simulink model "Motor_Pos_cl"  (R2015a)
settings: Solver=ode15s  StartTime=0.0  StopTime=10  RelTol=1e-3
values from neighbouring files (symbols this model uses):
  b = 3.5077E-6    (= 3.5077e-06)    [Motor_Pos_cl_m.m]
  J = 3.2284E-6    (= 3.2284e-06)    [Motor_Pos_cl_m.m]
  K = 0.0274    [Motor_Pos_cl_m.m]
  kd = 0    [Motor_Pos_cl_m.m]
  ki = 0    [Motor_Pos_cl_m.m]
  kp = 0.8    [Motor_Pos_cl_m.m]
  L = 2.75E-6    (= 2.75e-06)    [Motor_Pos_cl_m.m]
  R = 4    [Motor_Pos_cl_m.m]
  T1 = 0.040    (= 0.04)    [Motor_Pos_cl_m.m]
  T2 = 0.050    (= 0.05)    [Motor_Pos_cl_m.m]
libraries: simulink x2
settings Model: Creator=maen  LastModifiedBy=Xiaotian
settings DataIOCC: SignalLoggingSaveFormat=ModelDataLogs
settings OptimizationCC: ExpressionDepthLimit=2147483647
settings DebuggingCC: UnderspecifiedInitializationDetection=Classic  MergeDetectMultiDrivingBlocksExec=none  FcnCallInpInsideContextMsg=UseLocalSettings  StateNameClashWarn=warning
settings GRTTargetCC: CombineOutputUpdateFcns=off  GRTInterface=on

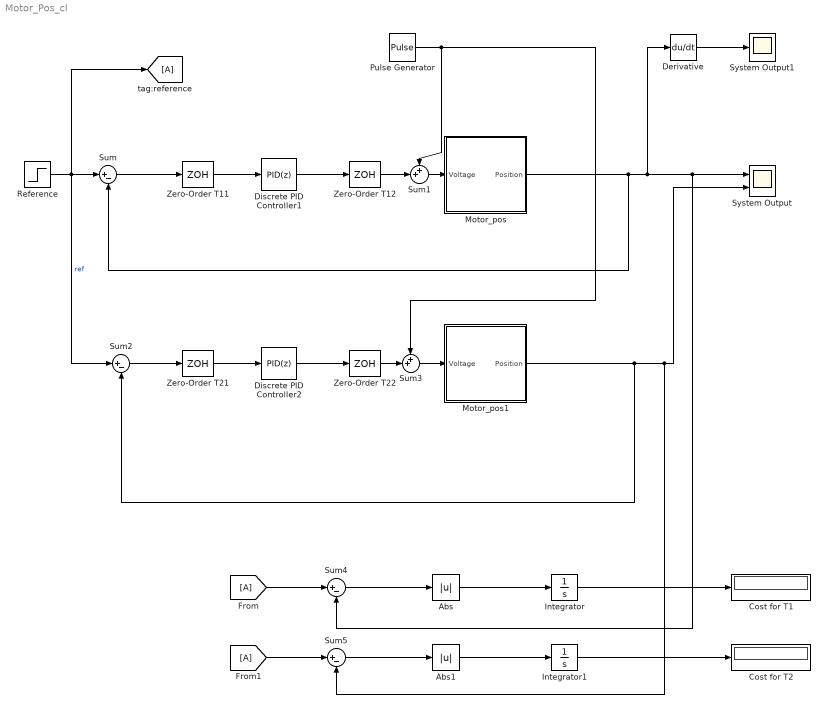
== system Motor_Pos_cl ==
  Abs : Abs
  Abs1 : Abs
  Cost for T1 : Display
  Cost for T2 : Display
  Derivative : Derivative
  Discrete PID Controller1 : simulink/Continuous/PID Controller  Controller=PID  TimeDomain=Discrete-time  SampleTime=T1  IntegratorMethod=Forward Euler  FilterMethod=Forward Euler  Form=Parallel  UseFilter=on  ControllerParametersSource=internal  P=kp  I=ki  D=kd  N=100  InitialConditionSource=internal  InitialConditionForIntegrator=0  InitialConditionForFilter=0  ExternalReset=none  LimitOutput=off  UpperSaturationLimit=inf  LowerSaturationLimit=-inf  LinearizeAsGain=off  AntiWindupMode=none  Kb=1  TrackingMode=off  Kt=1  PParamMin=[]  PParamMax=[]  IParamMin=[]  IParamMax=[]  DParamMin=[]  DParamMax=[]  NParamMin=[]  NParamMax=[]  KbParamMin=[]  KbParamMax=[]  KtParamMin=[]  KtParamMax=[]  POutMin=[]  POutMax=[]  IOutMin=[]  IOutMax=[]  DOutMin=[]  DOutMax=[]  NOutMin=[]  NOutMax=[]  KbOutMin=[]  KbOutMax=[]  KtOutMin=[]  KtOutMax=[]  IntegratorOutMin=[]  IntegratorOutMax=[]  FilterOutMin=[]  FilterOutMax=[]  SumOutMin=[]  SumOutMax=[]  SumI1OutMin=[]  SumI1OutMax=[]  SumI2OutMin=[]  SumI2OutMax=[]  SumI3OutMin=[]  SumI3OutMax=[]  SumDOutMin=[]  SumDOutMax=[]  SaturationOutMin=[]  SaturationOutMax=[]  IntegratorContinuousStateAttributes=''  IntegratorStateMustResolveToSignalObject=off  IntegratorRTWStateStorageClass=Auto  FilterContinuousStateAttributes=''  FilterStateMustResolveToSignalObject=off  FilterRTWStateStorageClass=Auto  DifferentiatorICPrevScaledInput=0  DifferentiatorOutMin=[]  DifferentiatorOutMax=[]
  Discrete PID Controller2 : simulink/Continuous/PID Controller  Controller=PID  TimeDomain=Discrete-time  SampleTime=T2  IntegratorMethod=Forward Euler  FilterMethod=Forward Euler  Form=Parallel  UseFilter=on  ControllerParametersSource=internal  P=kp  I=ki  D=kd  N=100  InitialConditionSource=internal  InitialConditionForIntegrator=0  InitialConditionForFilter=0  ExternalReset=none  LimitOutput=off  UpperSaturationLimit=inf  LowerSaturationLimit=-inf  LinearizeAsGain=off  AntiWindupMode=none  Kb=1  TrackingMode=off  Kt=1  PParamMin=[]  PParamMax=[]  IParamMin=[]  IParamMax=[]  DParamMin=[]  DParamMax=[]  NParamMin=[]  NParamMax=[]  KbParamMin=[]  KbParamMax=[]  KtParamMin=[]  KtParamMax=[]  POutMin=[]  POutMax=[]  IOutMin=[]  IOutMax=[]  DOutMin=[]  DOutMax=[]  NOutMin=[]  NOutMax=[]  KbOutMin=[]  KbOutMax=[]  KtOutMin=[]  KtOutMax=[]  IntegratorOutMin=[]  IntegratorOutMax=[]  FilterOutMin=[]  FilterOutMax=[]  SumOutMin=[]  SumOutMax=[]  SumI1OutMin=[]  SumI1OutMax=[]  SumI2OutMin=[]  SumI2OutMax=[]  SumI3OutMin=[]  SumI3OutMax=[]  SumDOutMin=[]  SumDOutMax=[]  SaturationOutMin=[]  SaturationOutMax=[]  IntegratorContinuousStateAttributes=''  IntegratorStateMustResolveToSignalObject=off  IntegratorRTWStateStorageClass=Auto  FilterContinuousStateAttributes=''  FilterStateMustResolveToSignalObject=off  FilterRTWStateStorageClass=Auto  DifferentiatorICPrevScaledInput=0  DifferentiatorOutMin=[]  DifferentiatorOutMax=[]
  Integrator : Integrator
  Integrator1 : Integrator
  Motor_pos : Subsystem
  Motor_pos1 : Subsystem
  Pulse Generator : DiscretePulseGenerator  PulseType=Time based  Amplitude=0.5  PulseWidth=2  PhaseDelay=2
  Reference : Step  Time=0  SampleTime=0
  Sum{,2,4..5} (4 alike) : Sum  Inputs=|+-
  Sum1 : Sum  Inputs=++|
  Sum3 : Sum  Inputs=++|
  System Output : Scope  NumInputPorts=2
      settings: TickLabels=on  TimeRange=15  YMin=0.967472~-5  YMax=1.03496~5  MaxDataPoints=10000
  System Output1 : Scope
      settings: YMin=1.0025  YMax=1.04  SaveName=ScopeData2
  Zero-Order T11 : ZeroOrderHold  SampleTime=T1
  Zero-Order T12 : ZeroOrderHold  SampleTime=T1
  Zero-Order T21 : ZeroOrderHold  SampleTime=T2
  Zero-Order T22 : ZeroOrderHold  SampleTime=T2
  wires:
  Reference/1 -> [A], Sum2/1, Sum/1  "ref"
  Sum/1 -> Zero-Order T11/1
  Zero-Order T11/1 -> Discrete PID Controller1/1
  Discrete PID Controller1/1 -> Zero-Order T12/1
  Derivative/1 -> System Output1/1
  Motor_pos/1(Position) -> System Output/1, Sum4/2, Derivative/1, Sum/2
  Pulse Generator/1 -> Sum3/1, Sum1/1
  Sum2/1 -> Zero-Order T21/1
  Zero-Order T21/1 -> Discrete PID Controller2/1
  Discrete PID Controller2/1 -> Zero-Order T22/1
  Motor_pos1/1(Position) -> Sum2/2, Sum5/2, System Output/2
  Integrator/1 -> Cost for T1/1
  Integrator1/1 -> Cost for T2/1
  Sum4/1 -> Abs/1
  [A] -> Sum4/1
  Abs/1 -> Integrator/1
  [A] -> Sum5/1
  Sum5/1 -> Abs1/1
  Abs1/1 -> Integrator1/1
  Sum1/1 -> Motor_pos/1(Voltage)
  Zero-Order T12/1 -> Sum1/2
  Zero-Order T22/1 -> Sum3/2
  Sum3/1 -> Motor_pos1/1(Voltage)

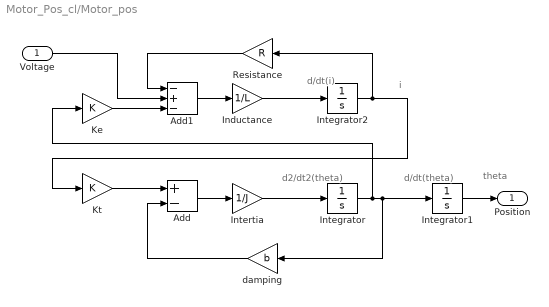
== system Motor_Pos_cl/Motor_pos ==
  note: i
  note: d/dt(theta)
  note: d2/dt2(theta)
  note: d/dt(i)
  note: theta
  Voltage : Inport
  Add : Sum  Inputs=+-
  Add1 : Sum  Inputs=-+-
  Inductance : Gain  Gain=1/L
  Integrator : Integrator
  Integrator1 : Integrator
  Integrator2 : Integrator
  Intertia : Gain  Gain=1/J
  Ke : Gain  Gain=K
  Kt : Gain  Gain=K
  Resistance : Gain  Gain=R
  damping : Gain  Gain=b
  Position : Outport
  wires:
  Inductance/1 -> Integrator2/1
  Integrator/1 -> Integrator1/1, damping/1, Ke/1
  Integrator1/1 -> Position/1
  Intertia/1 -> Integrator/1
  Integrator2/1 -> Kt/1, Resistance/1
  Add/1 -> Intertia/1
  Add1/1 -> Inductance/1
  Kt/1 -> Add/1
  damping/1 -> Add/2
  Ke/1 -> Add1/3
  Resistance/1 -> Add1/1
  Voltage/1 -> Add1/2

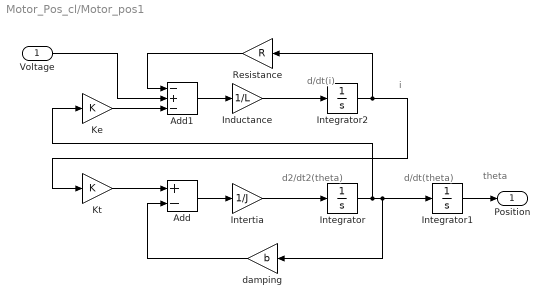
== system Motor_Pos_cl/Motor_pos1 ==
  note: i
  note: d/dt(theta)
  note: d2/dt2(theta)
  note: d/dt(i)
  note: theta
  Voltage : Inport
  Add : Sum  Inputs=+-
  Add1 : Sum  Inputs=-+-
  Inductance : Gain  Gain=1/L
  Integrator : Integrator
  Integrator1 : Integrator
  Integrator2 : Integrator
  Intertia : Gain  Gain=1/J
  Ke : Gain  Gain=K
  Kt : Gain  Gain=K
  Resistance : Gain  Gain=R
  damping : Gain  Gain=b
  Position : Outport
  wires:
  Inductance/1 -> Integrator2/1
  Integrator/1 -> Integrator1/1, damping/1, Ke/1
  Integrator1/1 -> Position/1
  Intertia/1 -> Integrator/1
  Integrator2/1 -> Kt/1, Resistance/1
  Add/1 -> Intertia/1
  Add1/1 -> Inductance/1
  Kt/1 -> Add/1
  damping/1 -> Add/2
  Ke/1 -> Add1/3
  Resistance/1 -> Add1/1
  Voltage/1 -> Add1/2
